simulink model "frequency_filter"  (R2023a)
settings: Solver=VariableStepAuto  StartTime=0.0  StopTime=tFinal  MaxStep=1/Fs  RelTol=1e-3
undefined symbols (not defined in the file or in its folder): gm, gphi, gw, kf
settings Model: Creator=Brandon Wright  LastModifiedBy=Brandon Wright

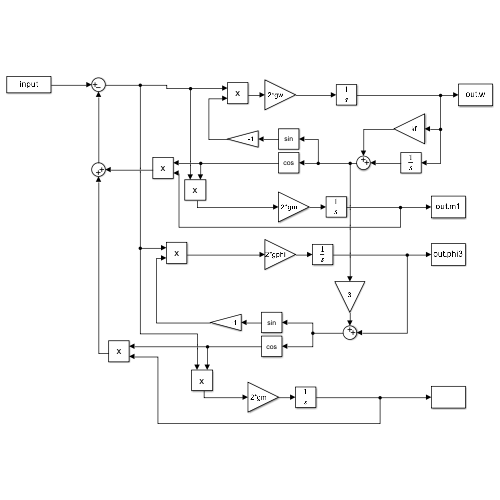
[thumbnail: Simulink's stored preview of the top-level diagram]
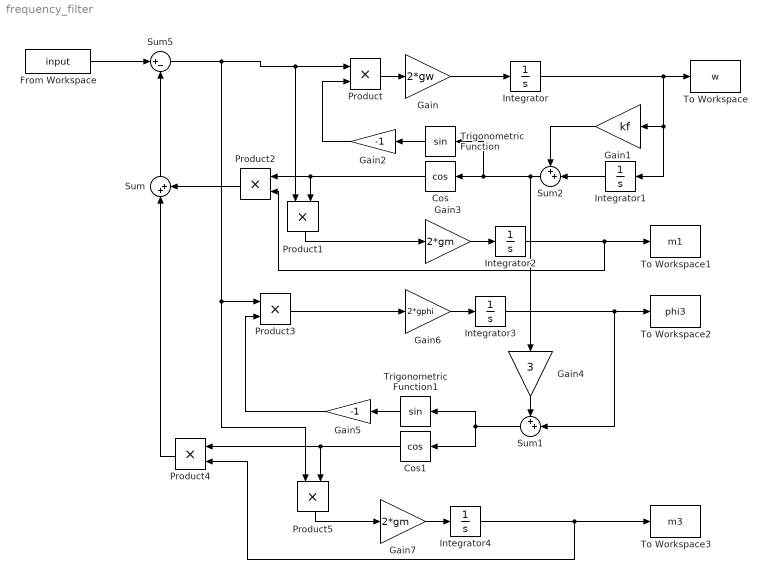
== system frequency_filter ==
  Cos : Trigonometry  Operator=cos
  Cos1 : Trigonometry  Operator=cos
  From Workspace : FromWorkspace  VariableName=input
  Gain : Gain  Gain=2*gw
  Gain1 : Gain  Gain=kf
  Gain2 : Gain  Gain=-1
  Gain3 : Gain  Gain=2*gm
  Gain4 : Gain  Gain=3
  Gain5 : Gain  Gain=-1
  Gain6 : Gain  Gain=2*gphi
  Gain7 : Gain  Gain=2*gm
  Integrator{,1..4} (5 alike) : Integrator
  Product{,1..5} (6 alike) : Product  RndMeth=Zero
  Sum : Sum  Inputs=|++
  Sum1 : Sum  Inputs=++|
  Sum2 : Sum  Inputs=++|
  Sum5 : Sum  Inputs=|+-
  To Workspace : ToWorkspace  VariableName=w  SampleTime=-1
  To Workspace1 : ToWorkspace  VariableName=m1  SampleTime=-1
  To Workspace2 : ToWorkspace  VariableName=phi3  SampleTime=-1
  To Workspace3 : ToWorkspace  VariableName=m3  SampleTime=-1
  Trigonometric Function : Trigonometry
  Trigonometric Function1 : Trigonometry
  wires:
  Gain/1 -> Integrator/1
  Integrator/1 -> Integrator1/1, Gain1/1, To Workspace/1
  Gain1/1 -> Sum2/1
  Integrator1/1 -> Sum2/2
  Trigonometric Function/1 -> Gain2/1
  Sum2/1 -> Cos/1, Trigonometric Function/1, Gain4/1
  Gain2/1 -> Product/2
  Product/1 -> Gain/1
  Product1/1 -> Gain3/1
  Cos/1 -> Product2/1, Product1/2
  Gain3/1 -> Integrator2/1
  Integrator2/1 -> Product2/2, To Workspace1/1
  Gain4/1 -> Sum1/1
  Trigonometric Function1/1 -> Gain5/1
  Sum1/1 -> Cos1/1, Trigonometric Function1/1
  Integrator3/1 -> Sum1/2, To Workspace2/1
  Gain6/1 -> Integrator3/1
  Product3/1 -> Gain6/1
  Gain5/1 -> Product3/2
  Product4/1 -> Sum/1
  Sum/1 -> Sum5/2
  Sum5/1 -> Product5/1, Product3/1, Product/1, Product1/1
  Product2/1 -> Sum/2
  Cos1/1 -> Product5/2, Product4/1
  Gain7/1 -> Integrator4/1
  Integrator4/1 -> Product4/2, To Workspace3/1
  Product5/1 -> Gain7/1
  From Workspace/1 -> Sum5/1
